simulink model "Relay_Auto_Tuning_R2015a"  (R2015a)
settings: Solver=ode3  SolverMode=SingleTasking  StartTime=t_start  StopTime=t_end  FixedStep=dt  MaxStep=1e-1  MinStep=1e-2  RelTol=1e-3
values from neighbouring files (symbols this model uses):
  d1 = 5    [Relay_Auto_Tuning_Procedure.m]    (also in Relay_Identification.m)
  d2 = 2    [Relay_Auto_Tuning_Procedure.m]    (also in Relay_Identification.m)
  Den = [10,10,10,1]    [Relay_Auto_Tuning_Procedure.m]
  h = 0.1    [Relay_Auto_Tuning_Procedure.m]    (also in Relay_Identification.m = min(d1,d2)*abs(dcgain(G))/mu)
  L = TF.OutputDelay    [AMIGO_Detune.m]    (also in AMIGO_Procedure.m = G.OutputDelay; AMIGO_Tune.m = 0.01; Benchmark_Decoupling_MIMO.m = 0.6*TNow; Benchmark_ModelError.m = 0.6*T)
  Num = 1    [Benchmark_Decoupling_MIMO.m]    (also in Benchmark_ModelError.m; Benchmark_ModelError_MIMO.m; Relay_Auto_Tuning_Procedure.m = [10,5])
  u0 = 2    [Relay_Auto_Tuning_Procedure.m]    (also in Relay_Identification.m = 10)
  y0 = dcgain(tf(Num,Den))*u0    [Relay_Auto_Tuning_Procedure.m]    (also in Relay_Identification.m = dcgain(G)*u0)
settings Model: CovMetricSettings=dwe  CovHtmlReporting=off  covSaveCumulativeToWorkspaceVar=off  CovSaveSingleToWorkspaceVar=off  CovExternalEMLEnable=on  Creator=juliu  LastModifiedBy=juliu
settings DataIOCC: LimitDataPoints=off  SaveFormat=Dataset
settings DebuggingCC: SFUnexpectedBacktrackingDiag=error  SFNoUnconditionalDefaultTransitionDiag=error
settings HardwareCC: ProdBitPerPointer=64  ProdLargestAtomicFloat=Float  ProdIntDivRoundTo=Zero  ProdEndianess=LittleEndian  ProdHWDeviceType=Specified
settings ModelReferenceCC: PropagateSignalLabelsOutOfModel=on
settings GRTTargetCC: TargetLangStandard=C99 (ISO)  GeneratePreprocessorConditionals=Use local settings

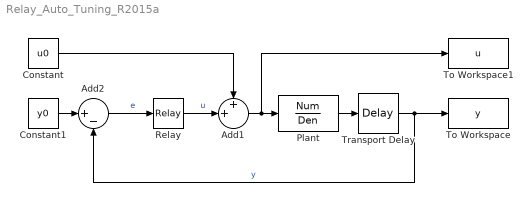
== system Relay_Auto_Tuning_R2015a ==
  Add1 : Sum  Inputs=++|
  Add2 : Sum  Inputs=|+-
  Constant : Constant  Value=u0
  Constant1 : Constant  Value=y0
  Plant : TransferFcn  Numerator=Num  Denominator=Den
  Relay : Relay  OnSwitchValue=h  OffSwitchValue=-h  OnOutputValue=+abs(d1)  OffOutputValue=-abs(d2)
  To Workspace : ToWorkspace  VariableName=y  SaveFormat=Timeseries  SampleTime=-1
  To Workspace1 : ToWorkspace  VariableName=u  SaveFormat=Timeseries  SampleTime=-1
  Transport Delay : TransportDelay  DelayTime=L  InitialOutput=y0
  wires:
  Plant/1 -> Transport Delay/1
  Relay/1 -> Add1/2  "u"
  Constant/1 -> Add1/1
  Add1/1 -> To Workspace1/1, Plant/1
  Transport Delay/1 -> Add2/2, To Workspace/1  "y"
  Add2/1 -> Relay/1  "e"
  Constant1/1 -> Add2/1
